simulink model "ADAS_Main"  (R2026a)
settings: Solver=FixedStepDiscrete  StopTime=5
InitFcn:
  | createLidarActorProfiles;
model workspace (MAT data in the model file):
  firstWarning = 1
  originalScenarioChecksum = '71EAF3DF157DF5A35F75811B676F8B0F'
undefined symbols (not defined in the file): driving, matlabshared
libraries: drivingscenarioandsensors x3, lidarlib x1
(part 1 of 6)
settings Model: Creator=sanga  LastModifiedBy=sanga
settings DebuggingCC: UnconnectedInputMsg=error

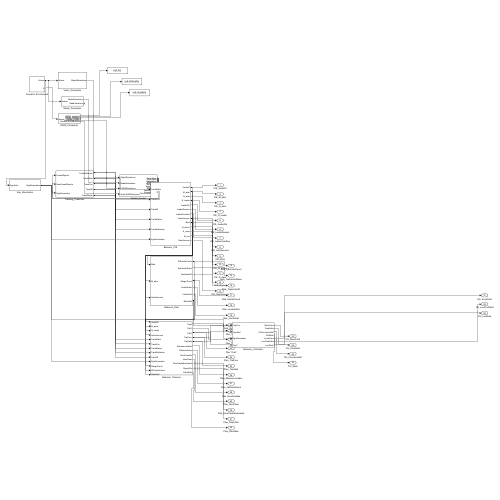
[thumbnail: Simulink's stored preview of the top-level diagram]
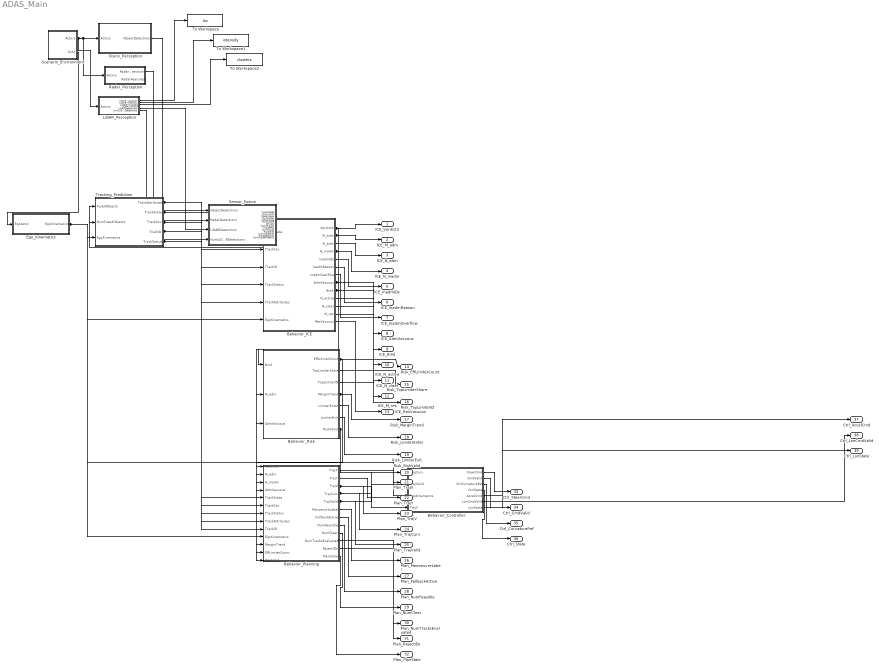
== system ADAS_Main ==
  Behavior_Controller : Subsystem
  Behavior_ICE : Subsystem
  Behavior_Planning : Subsystem
  Behavior_Risk : Subsystem
  Ego_Kinematics : Subsystem
  LiDAR_Perception : Subsystem
  Radar_Perception : Subsystem
  Scenario_Environment : Subsystem
  Sensor_Fusion : Subsystem
  To Workspace : ToWorkspace  VariableName=loc  SaveFormat=Timeseries  SampleTime=-1
  To Workspace1 : ToWorkspace  VariableName=intensity  SaveFormat=Timeseries  SampleTime=-1
  To Workspace2 : ToWorkspace  VariableName=clusters  SaveFormat=Timeseries  SampleTime=-1
  Tracking_Prediction : Subsystem
  Vision_Perception : Subsystem
  ICE_Verdict3 : Outport
  ICE_M_adm : Outport  Port=2
  ICE_N_adm : Outport  Port=3
  ICE_N_inadm : Outport  Port=4
  ICE_InadmIDs : Outport  Port=5
  ICE_InadmReason : Outport  Port=6
  ICE_InadmOverflow : Outport  Port=7
  ICE_AdmVacuous : Outport  Port=8
  ICE_Bind : Outport  Port=9
  ICE_N_active : Outport  Port=10
  ICE_N_clear : Outport  Port=11
  ICE_M_res : Outport  Port=12
  ICE_ResVacuous : Outport  Port=13
  Risk_EffLimiterCount : Outport  Port=14
  Risk_TopLimiterShare : Outport  Port=15
  Risk_TopLimiterID : Outport  Port=16
  Risk_MarginTrend : Outport  Port=17
  Risk_LimiterEnter : Outport  Port=18
  Risk_LimiterExit : Outport  Port=19
  Risk_RiskValid : Outport  Port=20
  Plan_TrajX : Outport  Port=21
  Plan_TrajY : Outport  Port=22
  Plan_TrajV : Outport  Port=23
  Plan_TrajCurv : Outport  Port=24
  Plan_TrajValid : Outport  Port=25
  Plan_ManoeuvreLabel : Outport  Port=26
  Plan_FallbackActive : Outport  Port=27
  Plan_NumFeasible : Outport  Port=28
  Plan_NumClear : Outport  Port=29
  Plan_NumTracksEvaluated : Outport  Port=30
  Plan_RejectIDs : Outport  Port=31
  Plan_PlanStale : Outport  Port=32
  Ctrl_SteerCmd : Outport  Port=33
  Ctrl_CmdValid : Outport  Port=34
  Ctrl_CurvatureRef : Outport  Port=35
  Ctrl_State : Outport  Port=36
  Ctrl_AccelCmd : Outport  Port=37
  Ctrl_LonCmdValid : Outport  Port=38
  Ctrl_LonState : Outport  Port=39
  wires:
  Scenario_Environment/1(Actors) -> Radar_Perception/1(Actors), Vision_Perception/1(Actors), LiDAR_Perception/1(Actors)
  LiDAR_Perception/1(LiDAR_Location) -> To Workspace/1
  LiDAR_Perception/2(LiDAR_Intensity) -> To Workspace1/1
  LiDAR_Perception/3(LiDAR_Clusters) -> To Workspace2/1
  Vision_Perception/1(ObjectDetections) -> Sensor_Fusion/1(ObjectDetections)
  Radar_Perception/1(RadarDetections) -> Sensor_Fusion/2(RadarDetections)
  LiDAR_Perception/5(LiDARDetections) -> Sensor_Fusion/3(LiDARDetections)
  LiDAR_Perception/6(NumLiDARDetections) -> Sensor_Fusion/4(NumLiDARDetections)
  Scenario_Environment/2(Out2) -> Ego_Kinematics/1(EgoActor)
  Sensor_Fusion/13(FusedObjects) -> Tracking_Prediction/1(FusedObjects)
  Sensor_Fusion/14(NumFusedObjects) -> Tracking_Prediction/2(NumFusedObjects)
  Ego_Kinematics/1(EgoKinematics) -> Tracking_Prediction/3(EgoKinematics), Behavior_ICE/6(EgoKinematics), Behavior_Planning/10(EgoKinematics), Behavior_Controller/3(EgoKinematics)
  Tracking_Prediction/2(TrackState) -> Behavior_ICE/1(TrackState), Behavior_Planning/5(TrackState)
  Tracking_Prediction/3(TrackCov) -> Behavior_ICE/2(TrackCov), Behavior_Planning/6(TrackCov)
  Tracking_Prediction/4(TrackID) -> Behavior_ICE/3(TrackID), Behavior_Planning/9(TrackID)
  Tracking_Prediction/5(TrackStatus) -> Behavior_ICE/4(TrackStatus), Behavior_Planning/7(TrackStatus)
  Tracking_Prediction/1(TrackAttributes) -> Behavior_ICE/5(TrackAttributes), Behavior_Planning/8(TrackAttributes)
  Behavior_ICE/1(Verdict3) -> ICE_Verdict3/1, Behavior_Planning/1(Verdict3)
  Behavior_ICE/2(M_adm) -> ICE_M_adm/1, Behavior_Risk/2(M_adm), Behavior_Planning/2(M_adm)
  Behavior_ICE/3(N_adm) -> ICE_N_adm/1
  Behavior_ICE/4(N_inadm) -> ICE_N_inadm/1, Behavior_Planning/3(N_inadm)
  Behavior_ICE/5(InadmIDs) -> ICE_InadmIDs/1
  Behavior_ICE/6(InadmReason) -> ICE_InadmReason/1
  Behavior_ICE/7(InadmOverflow) -> ICE_InadmOverflow/1
  Behavior_ICE/8(AdmVacuous) -> ICE_AdmVacuous/1, Behavior_Risk/3(AdmVacuous), Behavior_Planning/4(AdmVacuous)
  Behavior_ICE/9(Bind) -> ICE_Bind/1, Behavior_Risk/1(Bind)
  Behavior_ICE/10(N_active) -> ICE_N_active/1
  Behavior_ICE/11(N_clear) -> ICE_N_clear/1
  Behavior_ICE/12(M_res) -> ICE_M_res/1
  Behavior_ICE/13(ResVacuous) -> ICE_ResVacuous/1
  Behavior_Risk/1(EffLimiterCount) -> Risk_EffLimiterCount/1, Behavior_Planning/12(EffLimiterCount)
  Behavior_Risk/2(TopLimiterShare) -> Risk_TopLimiterShare/1
  Behavior_Risk/3(TopLimiterID) -> Risk_TopLimiterID/1
  Behavior_Risk/4(MarginTrend) -> Risk_MarginTrend/1, Behavior_Planning/11(MarginTrend)
  Behavior_Risk/5(LimiterEnter) -> Risk_LimiterEnter/1
  Behavior_Risk/6(LimiterExit) -> Risk_LimiterExit/1
  Behavior_Risk/7(RiskValid) -> Risk_RiskValid/1, Behavior_Planning/13(RiskValid)
  Behavior_Planning/1(TrajX) -> Plan_TrajX/1
  Behavior_Planning/2(TrajY) -> Plan_TrajY/1
  Behavior_Planning/3(TrajV) -> Plan_TrajV/1, Behavior_Controller/4(TrajV)
  Behavior_Planning/4(TrajCurv) -> Plan_TrajCurv/1, Behavior_Controller/1(TrajCurv)
  Behavior_Planning/5(TrajValid) -> Plan_TrajValid/1, Behavior_Controller/2(TrajValid)
  Behavior_Planning/6(ManoeuvreLabel) -> Plan_ManoeuvreLabel/1
  Behavior_Planning/7(FallbackActive) -> Plan_FallbackActive/1
  Behavior_Planning/8(NumFeasible) -> Plan_NumFeasible/1
  Behavior_Planning/9(NumClear) -> Plan_NumClear/1
  Behavior_Planning/10(NumTracksEvaluated) -> Plan_NumTracksEvaluated/1
  Behavior_Planning/11(RejectIDs) -> Plan_RejectIDs/1
  Behavior_Planning/12(PlanStale) -> Plan_PlanStale/1
  Behavior_Controller/1(SteerCmd) -> Ctrl_SteerCmd/1
  Behavior_Controller/2(CmdValid) -> Ctrl_CmdValid/1
  Behavior_Controller/3(CtrlCurvatureRef) -> Ctrl_CurvatureRef/1
  Behavior_Controller/4(CtrlState) -> Ctrl_State/1
  Behavior_Controller/5(AccelCmd) -> Ctrl_AccelCmd/1
  Behavior_Controller/6(LonCmdValid) -> Ctrl_LonCmdValid/1
  Behavior_Controller/7(LonState) -> Ctrl_LonState/1

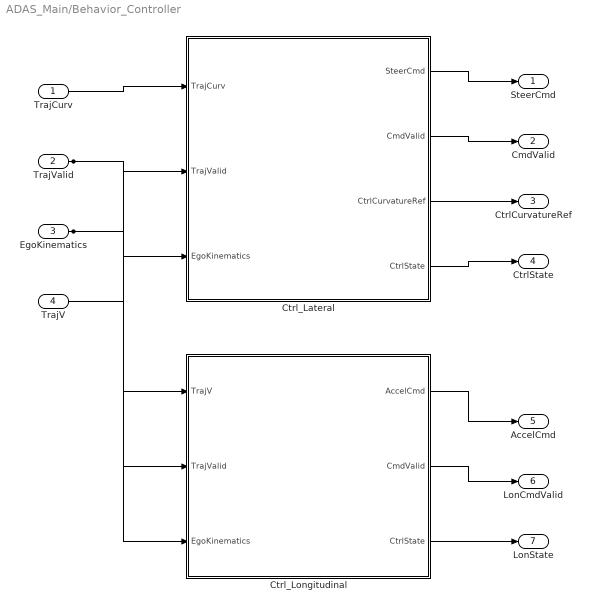
== system ADAS_Main/Behavior_Controller ==
  TrajCurv : Inport
  TrajValid : Inport  Port=2
  EgoKinematics : Inport  Port=3
  TrajV : Inport  Port=4
  Ctrl_Lateral : MATLAB Function  TreatAsAtomicUnit=on
  Ctrl_Longitudinal : MATLAB Function  TreatAsAtomicUnit=on
  SteerCmd : Outport
  CmdValid : Outport  Port=2
  CtrlCurvatureRef : Outport  Port=3
  CtrlState : Outport  Port=4
  AccelCmd : Outport  Port=5
  LonCmdValid : Outport  Port=6
  LonState : Outport  Port=7
  wires:
  TrajCurv/1 -> Ctrl_Lateral/1(TrajCurv)
  TrajValid/1 -> Ctrl_Lateral/2(TrajValid), Ctrl_Longitudinal/2(TrajValid)
  EgoKinematics/1 -> Ctrl_Lateral/3(EgoKinematics), Ctrl_Longitudinal/3(EgoKinematics)
  Ctrl_Lateral/1(SteerCmd) -> SteerCmd/1
  Ctrl_Lateral/2(CmdValid) -> CmdValid/1
  Ctrl_Lateral/3(CtrlCurvatureRef) -> CtrlCurvatureRef/1
  Ctrl_Lateral/4(CtrlState) -> CtrlState/1
  TrajV/1 -> Ctrl_Longitudinal/1(TrajV)
  Ctrl_Longitudinal/1(AccelCmd) -> AccelCmd/1
  Ctrl_Longitudinal/2(CmdValid) -> LonCmdValid/1
  Ctrl_Longitudinal/3(CtrlState) -> LonState/1

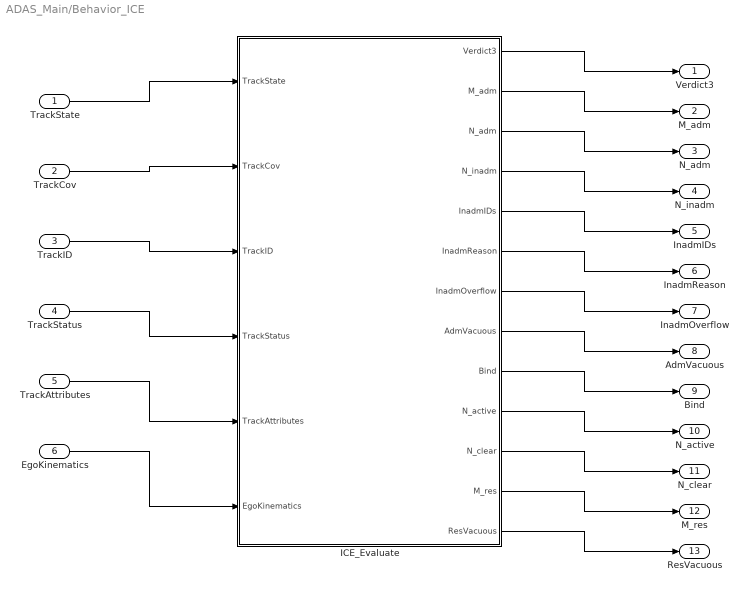
== system ADAS_Main/Behavior_ICE ==
  TrackState : Inport  OutDataTypeStr=double  PortDimensions=[512 4]
  TrackCov : Inport  Port=2  OutDataTypeStr=double  PortDimensions=[512 10]
  TrackID : Inport  Port=3  OutDataTypeStr=uint32  PortDimensions=[512 1]
  TrackStatus : Inport  Port=4  OutDataTypeStr=uint8  PortDimensions=[512 1]
  TrackAttributes : Inport  Port=5  OutDataTypeStr=double  PortDimensions=[512 4]
  EgoKinematics : Inport  Port=6  OutDataTypeStr=double  PortDimensions=[1 2]
  ICE_Evaluate : MATLAB Function  TreatAsAtomicUnit=on
  Verdict3 : Outport
  M_adm : Outport  Port=2
  N_adm : Outport  Port=3
  N_inadm : Outport  Port=4
  InadmIDs : Outport  Port=5
  InadmReason : Outport  Port=6
  InadmOverflow : Outport  Port=7
  AdmVacuous : Outport  Port=8
  Bind : Outport  Port=9
  N_active : Outport  Port=10
  N_clear : Outport  Port=11
  M_res : Outport  Port=12
  ResVacuous : Outport  Port=13
  wires:
  TrackState/1 -> ICE_Evaluate/1(TrackState)
  TrackCov/1 -> ICE_Evaluate/2(TrackCov)
  TrackID/1 -> ICE_Evaluate/3(TrackID)
  TrackStatus/1 -> ICE_Evaluate/4(TrackStatus)
  TrackAttributes/1 -> ICE_Evaluate/5(TrackAttributes)
  EgoKinematics/1 -> ICE_Evaluate/6(EgoKinematics)
  ICE_Evaluate/1(Verdict3) -> Verdict3/1
  ICE_Evaluate/2(M_adm) -> M_adm/1
  ICE_Evaluate/3(N_adm) -> N_adm/1
  ICE_Evaluate/4(N_inadm) -> N_inadm/1
  ICE_Evaluate/5(InadmIDs) -> InadmIDs/1
  ICE_Evaluate/6(InadmReason) -> InadmReason/1
  ICE_Evaluate/7(InadmOverflow) -> InadmOverflow/1
  ICE_Evaluate/8(AdmVacuous) -> AdmVacuous/1
  ICE_Evaluate/9(Bind) -> Bind/1
  ICE_Evaluate/10(N_active) -> N_active/1
  ICE_Evaluate/11(N_clear) -> N_clear/1
  ICE_Evaluate/12(M_res) -> M_res/1
  ICE_Evaluate/13(ResVacuous) -> ResVacuous/1

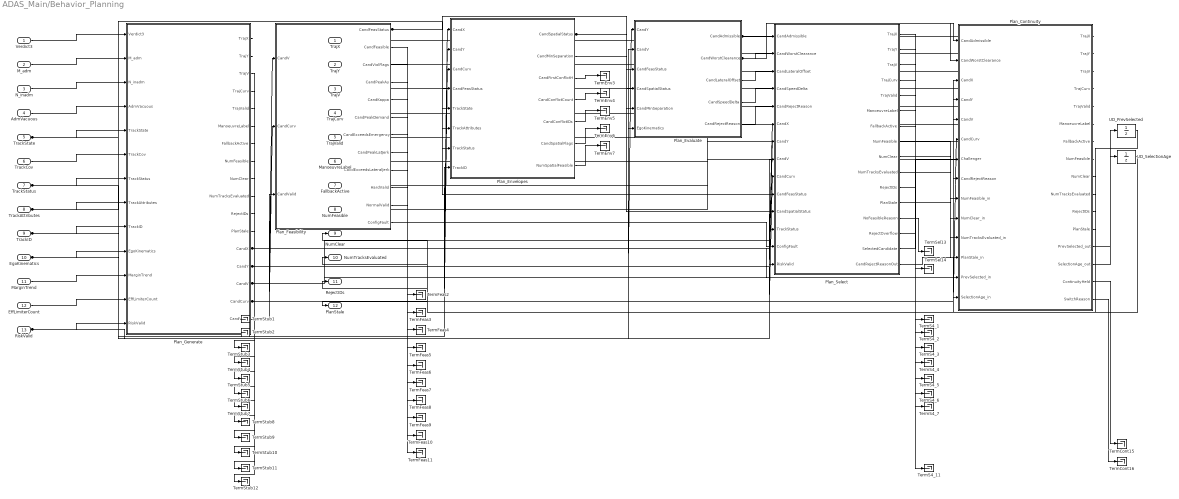
== system ADAS_Main/Behavior_Planning ==
  Verdict3 : Inport  OutDataTypeStr=int8  PortDimensions=[4 7]
  M_adm : Inport  Port=2  OutDataTypeStr=double  PortDimensions=[4 7]
  N_inadm : Inport  Port=3  OutDataTypeStr=uint16  PortDimensions=[1 1]
  AdmVacuous : Inport  Port=4  OutDataTypeStr=boolean  PortDimensions=[1 1]
  TrackState : Inport  Port=5  OutDataTypeStr=double  PortDimensions=[512 4]
  TrackCov : Inport  Port=6  OutDataTypeStr=double  PortDimensions=[512 10]
  TrackStatus : Inport  Port=7  OutDataTypeStr=uint8  PortDimensions=[512 1]
  TrackAttributes : Inport  Port=8  OutDataTypeStr=double  PortDimensions=[512 4]
  TrackID : Inport  Port=9  OutDataTypeStr=uint32  PortDimensions=[512 1]
  EgoKinematics : Inport  Port=10  OutDataTypeStr=double  PortDimensions=[1 2]
  MarginTrend : Inport  Port=11  OutDataTypeStr=double  PortDimensions=[4 7]
  EffLimiterCount : Inport  Port=12  OutDataTypeStr=double  PortDimensions=[4 1]
  RiskValid : Inport  Port=13  OutDataTypeStr=boolean  PortDimensions=[1 1]
  Plan_Continuity : MATLAB Function  TreatAsAtomicUnit=on
  Plan_Envelopes : MATLAB Function  TreatAsAtomicUnit=on
  Plan_Evaluate : MATLAB Function  TreatAsAtomicUnit=on
  Plan_Feasibility : MATLAB Function  TreatAsAtomicUnit=on
  Plan_Generate : MATLAB Function  TreatAsAtomicUnit=on
  Plan_Select : MATLAB Function  TreatAsAtomicUnit=on
  TermCont15 : Terminator
  TermCont16 : Terminator
  TermEnv{3..7} (5 alike) : Terminator
  TermFeas{2..11} (10 alike) : Terminator
  TermS4_{1..7,11} (8 alike) : Terminator
  TermSel13 : Terminator
  TermSel14 : Terminator
  TermStub{1..12} (12 alike) : Terminator
  UD_PrevSelected : UnitDelay  SampleTime=-1
  UD_SelectionAge : UnitDelay  SampleTime=-1
  TrajX : Outport
  TrajY : Outport  Port=2
  TrajV : Outport  Port=3
  TrajCurv : Outport  Port=4
  TrajValid : Outport  Port=5
  ManoeuvreLabel : Outport  Port=6
  FallbackActive : Outport  Port=7
  NumFeasible : Outport  Port=8
  NumClear : Outport  Port=9
  NumTracksEvaluated : Outport  Port=10
  RejectIDs : Outport  Port=11
  PlanStale : Outport  Port=12
  wires:
  Verdict3/1 -> Plan_Generate/1(Verdict3)
  M_adm/1 -> Plan_Generate/2(M_adm)
  N_inadm/1 -> Plan_Generate/3(N_inadm)
  AdmVacuous/1 -> Plan_Generate/4(AdmVacuous)
  TrackState/1 -> Plan_Generate/5(TrackState), Plan_Envelopes/5(TrackState)
  TrackCov/1 -> Plan_Generate/6(TrackCov)
  TrackStatus/1 -> Plan_Generate/7(TrackStatus), Plan_Envelopes/7(TrackStatus), Plan_Select/12(TrackStatus)
  TrackAttributes/1 -> Plan_Generate/8(TrackAttributes), Plan_Envelopes/6(TrackAttributes)
  TrackID/1 -> Plan_Generate/9(TrackID), Plan_Envelopes/8(TrackID)
  EgoKinematics/1 -> Plan_Generate/10(EgoKinematics), Plan_Evaluate/6(EgoKinematics)
  MarginTrend/1 -> Plan_Generate/11(MarginTrend)
  EffLimiterCount/1 -> Plan_Generate/12(EffLimiterCount)
  RiskValid/1 -> Plan_Generate/13(RiskValid), Plan_Select/14(RiskValid)
  Plan_Generate/15(CandV) -> Plan_Feasibility/1(CandV), Plan_Evaluate/2(CandV), Plan_Select/8(CandV), Plan_Continuity/5(CandV)
  Plan_Generate/16(CandCurv) -> Plan_Feasibility/2(CandCurv), Plan_Envelopes/3(CandCurv), Plan_Select/9(CandCurv), Plan_Continuity/6(CandCurv)
  Plan_Generate/17(CandValid) -> Plan_Feasibility/3(CandValid)
  Plan_Feasibility/2(CandFeasible) -> TermFeas2/1
  Plan_Feasibility/3(CandViolFlags) -> TermFeas3/1
  Plan_Feasibility/4(CandPeakAy) -> TermFeas4/1
  Plan_Feasibility/5(CandKappa) -> TermFeas5/1
  Plan_Feasibility/6(CandPeakDemand) -> TermFeas6/1
  Plan_Feasibility/7(CandExceedsEmergency) -> TermFeas7/1
  Plan_Feasibility/8(CandPeakLatJerk) -> TermFeas8/1
  Plan_Feasibility/9(CandExceedsLateralJerk) -> TermFeas9/1
  Plan_Feasibility/10(HardValid) -> TermFeas10/1
  Plan_Feasibility/11(NormalValid) -> TermFeas11/1
  Plan_Generate/13(CandX) -> Plan_Envelopes/1(CandX), Plan_Select/6(CandX), Plan_Continuity/3(CandX)
  Plan_Generate/14(CandY) -> Plan_Envelopes/2(CandY), Plan_Evaluate/1(CandY), Plan_Select/7(CandY), Plan_Continuity/4(CandY)
  Plan_Feasibility/1(CandFeasStatus) -> Plan_Envelopes/4(CandFeasStatus), Plan_Evaluate/3(CandFeasStatus), Plan_Select/10(CandFeasStatus)
  Plan_Envelopes/3(CandFirstConflictH) -> TermEnv3/1
  Plan_Envelopes/4(CandConflictCount) -> TermEnv4/1
  Plan_Envelopes/5(CandConflictIDs) -> TermEnv5/1
  Plan_Envelopes/6(CandSpatialFlags) -> TermEnv6/1
  Plan_Envelopes/7(NumSpatialFeasible) -> TermEnv7/1
  Plan_Generate/1(TrajX) -> TermStub1/1
  Plan_Generate/2(TrajY) -> TermStub2/1
  Plan_Generate/3(TrajV) -> TermStub3/1
  Plan_Generate/4(TrajCurv) -> TermStub4/1
  Plan_Generate/5(TrajValid) -> TermStub5/1
  Plan_Generate/6(ManoeuvreLabel) -> TermStub6/1
  Plan_Generate/7(FallbackActive) -> TermStub7/1
  Plan_Generate/8(NumFeasible) -> TermStub8/1
  Plan_Generate/9(NumClear) -> TermStub9/1
  Plan_Generate/10(NumTracksEvaluated) -> TermStub10/1
  Plan_Generate/11(RejectIDs) -> TermStub11/1
  Plan_Generate/12(PlanStale) -> TermStub12/1
  Plan_Envelopes/1(CandSpatialStatus) -> Plan_Evaluate/4(CandSpatialStatus), Plan_Select/11(CandSpatialStatus)
  Plan_Envelopes/2(CandMinSeparation) -> Plan_Evaluate/5(CandMinSeparation)
  Plan_Evaluate/1(CandAdmissible) -> Plan_Select/1(CandAdmissible), Plan_Continuity/1(CandAdmissible)
  Plan_Evaluate/2(CandWorstClearance) -> Plan_Select/2(CandWorstClearance), Plan_Continuity/2(CandWorstClearance)
  Plan_Evaluate/3(CandLateralOffset) -> Plan_Select/3(CandLateralOffset)
  Plan_Evaluate/4(CandSpeedDelta) -> Plan_Select/4(CandSpeedDelta)
  Plan_Evaluate/5(CandRejectReason) -> Plan_Select/5(CandRejectReason)
  Plan_Feasibility/12(ConfigFault) -> Plan_Select/13(ConfigFault)
  Plan_Select/13(NoFeasibleReason) -> TermSel13/1
  Plan_Select/14(RejectOverflow) -> TermSel14/1
  Plan_Select/15(SelectedCandidate) -> Plan_Continuity/7(Challenger)
  Plan_Select/16(CandRejectReasonOut) -> Plan_Continuity/8(CandRejectReason)
  Plan_Select/8(NumFeasible) -> Plan_Continuity/9(NumFeasible_in)
  Plan_Select/9(NumClear) -> Plan_Continuity/10(NumClear_in)
  Plan_Select/10(NumTracksEvaluated) -> Plan_Continuity/11(NumTracksEvaluated_in)
  Plan_Select/12(PlanStale) -> Plan_Continuity/12(PlanStale_in)
  UD_PrevSelected/1 -> Plan_Continuity/13(PrevSelected_in)
  UD_SelectionAge/1 -> Plan_Continuity/14(SelectionAge_in)
  Plan_Continuity/1(TrajX) -> TrajX/1
  Plan_Continuity/2(TrajY) -> TrajY/1
  Plan_Continuity/3(TrajV) -> TrajV/1
  Plan_Continuity/4(TrajCurv) -> TrajCurv/1
  Plan_Continuity/5(TrajValid) -> TrajValid/1
  Plan_Continuity/6(ManoeuvreLabel) -> ManoeuvreLabel/1
  Plan_Continuity/7(FallbackActive) -> FallbackActive/1
  Plan_Continuity/8(NumFeasible) -> NumFeasible/1
  Plan_Continuity/9(NumClear) -> NumClear/1
  Plan_Continuity/10(NumTracksEvaluated) -> NumTracksEvaluated/1
  Plan_Continuity/11(RejectIDs) -> RejectIDs/1
  Plan_Continuity/12(PlanStale) -> PlanStale/1
  Plan_Continuity/13(PrevSelected_out) -> UD_PrevSelected/1
  Plan_Continuity/14(SelectionAge_out) -> UD_SelectionAge/1
  Plan_Continuity/15(ContinuityHeld) -> TermCont15/1
  Plan_Continuity/16(SwitchReason) -> TermCont16/1
  Plan_Select/1(TrajX) -> TermS4_1/1
  Plan_Select/2(TrajY) -> TermS4_2/1
  Plan_Select/3(TrajV) -> TermS4_3/1
  Plan_Select/4(TrajCurv) -> TermS4_4/1
  Plan_Select/5(TrajValid) -> TermS4_5/1
  Plan_Select/6(ManoeuvreLabel) -> TermS4_6/1
  Plan_Select/7(FallbackActive) -> TermS4_7/1
  Plan_Select/11(RejectIDs) -> TermS4_11/1

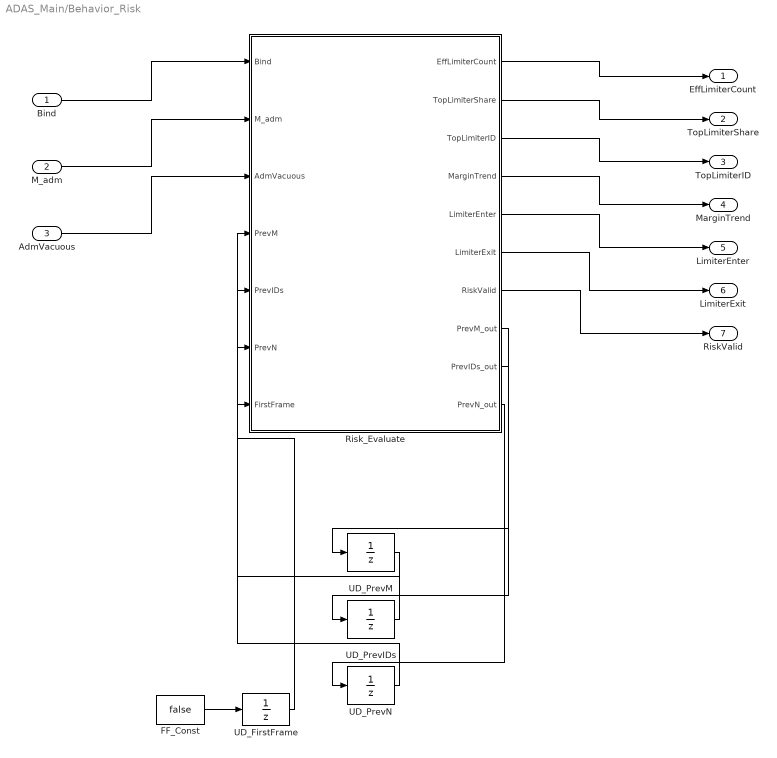
== system ADAS_Main/Behavior_Risk ==
  Bind : Inport  OutDataTypeStr=uint32  PortDimensions=[4 7 8]
  M_adm : Inport  Port=2  OutDataTypeStr=double  PortDimensions=[4 7]
  AdmVacuous : Inport  Port=3  OutDataTypeStr=boolean  PortDimensions=[1 1]
  FF_Const : Constant  Value=false  OutDataTypeStr=boolean
  Risk_Evaluate : MATLAB Function  TreatAsAtomicUnit=on
  UD_FirstFrame : UnitDelay  InitialCondition=1  SampleTime=0.1
  UD_PrevIDs : UnitDelay  SampleTime=0.1
  UD_PrevM : UnitDelay  SampleTime=0.1
  UD_PrevN : UnitDelay  SampleTime=0.1
  EffLimiterCount : Outport
  TopLimiterShare : Outport  Port=2
  TopLimiterID : Outport  Port=3
  MarginTrend : Outport  Port=4
  LimiterEnter : Outport  Port=5
  LimiterExit : Outport  Port=6
  RiskValid : Outport  Port=7
  wires:
  Bind/1 -> Risk_Evaluate/1(Bind)
  M_adm/1 -> Risk_Evaluate/2(M_adm)
  AdmVacuous/1 -> Risk_Evaluate/3(AdmVacuous)
  Risk_Evaluate/8(PrevM_out) -> UD_PrevM/1
  UD_PrevM/1 -> Risk_Evaluate/4(PrevM)
  Risk_Evaluate/9(PrevIDs_out) -> UD_PrevIDs/1
  UD_PrevIDs/1 -> Risk_Evaluate/5(PrevIDs)
  Risk_Evaluate/10(PrevN_out) -> UD_PrevN/1
  UD_PrevN/1 -> Risk_Evaluate/6(PrevN)
  FF_Const/1 -> UD_FirstFrame/1
  UD_FirstFrame/1 -> Risk_Evaluate/7(FirstFrame)
  Risk_Evaluate/1(EffLimiterCount) -> EffLimiterCount/1
  Risk_Evaluate/2(TopLimiterShare) -> TopLimiterShare/1
  Risk_Evaluate/3(TopLimiterID) -> TopLimiterID/1
  Risk_Evaluate/4(MarginTrend) -> MarginTrend/1
  Risk_Evaluate/5(LimiterEnter) -> LimiterEnter/1
  Risk_Evaluate/6(LimiterExit) -> LimiterExit/1
  Risk_Evaluate/7(RiskValid) -> RiskValid/1

== system ADAS_Main/Ego_Kinematics ==
  EgoActor : Inport
  Extract_Ego_Kinematics : MATLAB Function  TreatAsAtomicUnit=on
  TW_EgoKin : ToWorkspace  VariableName=egoKin  SaveFormat=Timeseries  SampleTime=-1
  EgoKinematics : Outport
  wires:
  EgoActor/1 -> Extract_Ego_Kinematics/1(egoActor)
  Extract_Ego_Kinematics/1(egoKin) -> EgoKinematics/1, TW_EgoKin/1

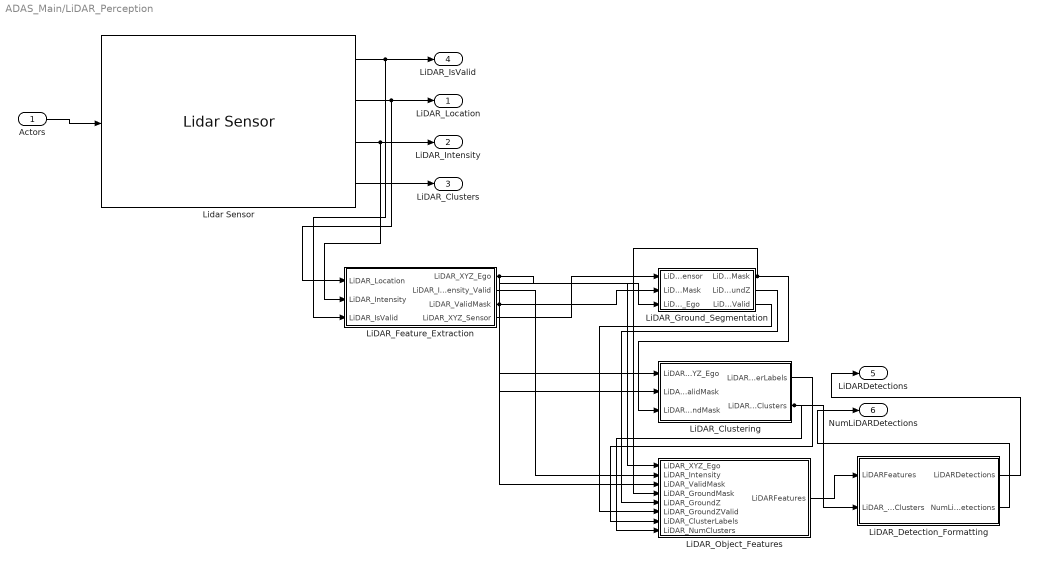
== system ADAS_Main/LiDAR_Perception ==
  Actors : Inport
  LiDAR_Clustering : Subsystem
  LiDAR_Detection_Formatting : Subsystem
  LiDAR_Feature_Extraction : Subsystem
  LiDAR_Ground_Segmentation : Subsystem
  LiDAR_Object_Features : Subsystem
  Lidar Sensor : lidarlib/Lidar Sensor  SensorIndex=1  UpdateRate=0.1  Model=Custom  SensorPosition=[1.5 0 1.6]  SensorOrientation=[0 0 0]  ActorProfilesVariableName=actor_profiles  HostID=1  CoordinateSystem=Sensor  MaxRange=120  AzimuthLimits=[-180 180]  AzimuthResolution=0.16  UseCustomElevationAngles=off  ElevationAngles=[-25 -15.6 -11.3 -8.8:0.9:-4 -4:0.32:1.6 3.3 4.6 7 10.3 15]  ElevationLimits=[-20 20]  ElevationResolution=0.4  HasNoise=on  RangeAccuracy=0.01  FogVisibility=1000  Rainrate=0  HasMotionDistortion=off  FiringTimes=[]  MaterialAttributesJSON=|  EditMaterialAttributesJSON=off  OutputIntensity=on  OutputClusters=on
      | [
      | {"Material":"Aluminum","Reflectance":0.63,"Diffuseness":1,"Roughness":0.3,"Description":"Weathered aluminum metal from roof"},
      | {"Material":"Asphalt","Reflectance":0.1,"Diffuseness":1,"Roughness":0.3,"Description":"Road or construction material"},
      | {"Material":"Bark","Reflectance":0.56,"Diffuseness":1,"Roughness":0.3,"Description":"Pinus ponderosa tree bark"},
      | {"Material":"Brick","Reflectance":0.29,"Diffuseness":1,"Roughness":0.3,"Description":"Smooth-faced red building construction brick"},
      | {"Material":"Cement","Reflectance":0.35,"Diffuseness":1,"Roughness":0.3,"Description":"Cement construction concrete cinderblock"},
      | {"Material":"Concrete","Reflectance":0.33,"Diffuseness":1,"Roughness":0.3,"Description":"Road or construction material"},
      | {"Material":"Copper","Reflectance":0.57,"Diffuseness":1,"Roughness":0.3,"Description":"Weathered copper metal from roof"},
      | {"Material":"Default","Reflectance":1,"Diffuseness":1,"Roughness":0.3,"Description":"Default material attributes"},
      | {"Material":"Glass","Reflectance":0.08,"Diffuseness":1,"Roughness":0.3,"Description":"Transparent construction plate window glass"},
      | {"Material":"Grass","Reflectance":0.5,"Diffuseness":1,"Roughness":0.3,"Description":"Green Rye grass"},
      | {"Material":"Ice","Reflectance":0.017,"Diffuseness":1,"Roughness":0.3,"Description":"Ice"},
      | {"Material":"Leaves","Reflectance":0.56,"Diffuseness":1,"Roughness":0.3,"Description":"Quercus species (Oak tree) leaves"},
      | {"Material":"Marble","Reflectance":0.84,"Diffuseness":1,"Roughness":0.3,"Description":"White weathered construction marble"},
      | {"Material":"Rubber","Reflectance":0.6,"Diffuseness":1,"Roughness":0.3,"Description":"White rubberized coating from building roof"},
      | {"Material":"Snow","Reflectance":0.71,"Diffuseness":1,"Roughness":0.3,"Description":"Coarse granular snow"},
      | {"Material":"Steel","Reflectance":0.064,"Diffuseness":1,"Roughness":0.3,"Description":"Weathered, galvanized steel metal from roof"},
      | {"Material":"Tar","Reflectance":0.07,"Diffuseness":1,"Roughness":0.3,"Description":"Black, glossy construction tar"},
      | {"Material":"Terracotta","Reflectance":0.17,"Diffuseness":1,"Roughness":0.3,"Description":"Weathered terra cotta roofing tile of ceramic composite construction"},
      | {"Material":"Water","Reflectance":0.025,"Diffuseness":1,"Roughness":0.3,"Description":"Tap water"},
      | {"Material":"Wood","Reflectance":0.85,"Diffuseness":1,"Roughness":0.3,"Description":"Bare pine wood construction lumber"}
      | ]
  LiDAR_Location : Outport
  LiDAR_Intensity : Outport  Port=2
  LiDAR_Clusters : Outport  Port=3
  LiDAR_IsValid : Outport  Port=4
  LiDARDetections : Outport  Port=5
  NumLiDARDetections : Outport  Port=6
  wires:
  Lidar Sensor/2 -> LiDAR_Feature_Extraction/1(LiDAR_Location), LiDAR_Location/1
  Lidar Sensor/3 -> LiDAR_Feature_Extraction/2(LiDAR_Intensity), LiDAR_Intensity/1
  Lidar Sensor/4 -> LiDAR_Clusters/1
  Lidar Sensor/1 -> LiDAR_Feature_Extraction/3(LiDAR_IsValid), LiDAR_IsValid/1
  LiDAR_Feature_Extraction/4(LiDAR_XYZ_Sensor) -> LiDAR_Ground_Segmentation/1(LiDAR_XYZ_Sensor)
  LiDAR_Feature_Extraction/3(LiDAR_ValidMask) -> LiDAR_Ground_Segmentation/2(LiDAR_ValidMask), LiDAR_Clustering/2(LiDAR_ValidMask), LiDAR_Object_Features/3(LiDAR_ValidMask)
  Actors/1 -> Lidar Sensor/1
  LiDAR_Feature_Extraction/1(LiDAR_XYZ_Ego) -> LiDAR_Ground_Segmentation/3(LiDAR_XYZ_Ego), LiDAR_Clustering/1(LiDAR_XYZ_Ego), LiDAR_Object_Features/1(LiDAR_XYZ_Ego)
  LiDAR_Ground_Segmentation/1(LiDAR_GroundMask) -> LiDAR_Clustering/3(LiDAR_GroundMask), LiDAR_Object_Features/4(LiDAR_GroundMask)
  LiDAR_Feature_Extraction/2(LiDAR_Intensity_Valid) -> LiDAR_Object_Features/2(LiDAR_Intensity)
  LiDAR_Ground_Segmentation/2(LiDAR_GroundZ) -> LiDAR_Object_Features/5(LiDAR_GroundZ)
  LiDAR_Ground_Segmentation/3(LiDAR_GroundZValid) -> LiDAR_Object_Features/6(LiDAR_GroundZValid)
  LiDAR_Clustering/1(LiDAR_ClusterLabels) -> LiDAR_Object_Features/7(LiDAR_ClusterLabels)
  LiDAR_Clustering/2(LiDAR_NumClusters) -> LiDAR_Object_Features/8(LiDAR_NumClusters), LiDAR_Detection_Formatting/2(LiDAR_NumClusters)
  LiDAR_Object_Features/1(LiDARFeatures) -> LiDAR_Detection_Formatting/1(LiDARFeatures)
  LiDAR_Detection_Formatting/1(LiDARDetections) -> LiDARDetections/1
  LiDAR_Detection_Formatting/2(NumLiDARDetections) -> NumLiDARDetections/1

== system ADAS_Main/Radar_Perception ==
  Actors : Inport
  Driving Radar Data Generator : drivingscenarioandsensors/Driving Radar Data Generator  SensorIndex=2  UpdateRate=10  MountingLocation=[ 3.4, 0, 0.2 ]  MountingAngles=[0 0 0]  HasElevation=off  HasRangeRate=on  HasNoise=on  HasFalseAlarms=on  HasOcclusion=on  MaxNumReportsSource=Property  MaxNumReports=50  TargetReportFormat=Clustered detections  DetectionCoordinates=Body  TrackCoordinates=Body  BusNameSource=Auto  BusName=BusDrivingRadarDataGenerator  SimulateUsing=Interpreted execution  AzimuthResolution=4  ElevationResolution=5  RangeResolution=2.5  RangeRateResolution=0.5  AzimuthBiasFraction=0.1  ElevationBiasFraction=0.1  RangeBiasFraction=0.05  RangeRateBiasFraction=0.05  FieldOfView=[ 20, 5 ]  RangeLimits=[ 0, 150 ]  RangeRateLimits=[ -100, 100 ]  DetectionProbability=0.9  FalseAlarmRate=1e-06  ReferenceRange=100  ReferenceRCS=0  CenterFrequency=77e9  FilterInitializationFcn=initcvekf  ConfirmationThreshold=[2 3]  DeletionThreshold=[5 5]  InitialSeedSource=Repeatable  InitialSeed=0  UsedSeed=matlabshared.tracking.internal.SimulinkUtilities.seedManager(gcb)  ProfilesSource=From Scenario Reader block  ProfilesParameters=driving.internal.ActorProfilesRadarParameters  ProfilesExpression=struct('ClassID',0,'Length',4.7,'Width',1.8,'Height',1.4,'OriginOffset',[-1.35 0 0],'RCSPattern',[10 10;10 10],'RCSAzimuthAngles',[-180 180],'RCSElevationAngles',[-90 90])
  Radar_Feature_Extraction : Subsystem
  RadarDetections : Outport
  RadarFeatures : Outport  Port=2
  wires:
  Actors/1 -> Driving Radar Data Generator/1
  Driving Radar Data Generator/1 -> Radar_Feature_Extraction/1(RawRadarDetections)
  Radar_Feature_Extraction/1(EnhancedRadar) -> RadarDetections/1
  Radar_Feature_Extraction/2(RadarFeatures) -> RadarFeatures/1

== system ADAS_Main/Scenario_Environment ==
  Bus Selector : BusSelector  OutputSignals=Position,Velocity
  Scenario Reader : drivingscenarioandsensors/Scenario Reader  Priority=-1  ScenarioSource=From file  ScenarioFileName=D:\AutonomousDriving\D_scenarios\V2_0_CameraScenario.mat  ScenarioVariableName=scenario  OutputCoordinateSystem=Vehicle coordinates  EgoVehicleSource=Scenario  EgoVehicleActorID=1  OrientVehiclesOnRoad=off  OutputEgoVehiclePose=on  OutputEgoVehicleState=on  SampleTime=0.1  LaneBoundaryOutput=None  LaneBoundaryDistance=0:0.5:9.5  LaneBoundaryLocation=Center of lane markings  BusNameSource=Auto  BusName=BusActors  BusNumActorsSource=Scenario  BusNumActors=100  BusName2Source=Auto  BusName2=BusLaneBoundaries  BusNumLaneBoundariesSource=Scenario  BusNumLaneBoundaries=10  BusName3Source=Auto  BusName3=BusEgoActor  BusName4Source=Auto  BusName4=BusEgoState  ShowCoordinateLabels=on  SimulateUsing=Interpreted execution
  Scope : Scope
      settings: ActiveDisplayYMinimum=-16.478455804620214  ActiveDisplayYMaximum=59.403600827046532
  Scope1 : Scope
      settings: ActiveDisplayYMinimum=-0.75912369165439664  ActiveDisplayYMaximum=11.206530935880661
  Actors : Outport
  Out2 : Outport  Port=2
  wires:
  Bus Selector/2 -> Scope1/1  "<Velocity>"
  Scenario Reader/3 -> Bus Selector/1
  Scenario Reader/1 -> Actors/1
  Scenario Reader/2 -> Out2/1
  Bus Selector/1 -> Scope/1  "<Position>"

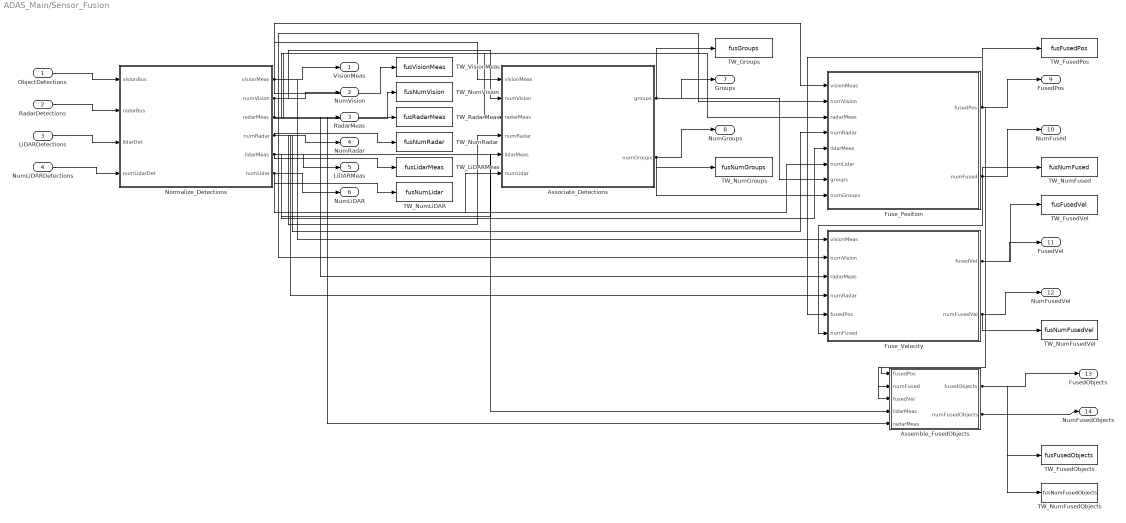
== system ADAS_Main/Sensor_Fusion ==
  ObjectDetections : Inport
  RadarDetections : Inport  Port=2
  LiDARDetections : Inport  Port=3
  NumLiDARDetections : Inport  Port=4
  Assemble_FusedObjects : MATLAB Function  TreatAsAtomicUnit=on
  Associate_Detections : MATLAB Function  TreatAsAtomicUnit=on
  Fuse_Position : MATLAB Function  TreatAsAtomicUnit=on
  Fuse_Velocity : MATLAB Function  TreatAsAtomicUnit=on
  Normalize_Detections : MATLAB Function  TreatAsAtomicUnit=on
  TW_FusedObjects : ToWorkspace  VariableName=fusFusedObjects  SaveFormat=Timeseries  SampleTime=-1
  TW_FusedPos : ToWorkspace  VariableName=fusFusedPos  SaveFormat=Timeseries  SampleTime=-1
  TW_FusedVel : ToWorkspace  VariableName=fusFusedVel  SaveFormat=Timeseries  SampleTime=-1
  TW_Groups : ToWorkspace  VariableName=fusGroups  SaveFormat=Timeseries  SampleTime=-1
  TW_LiDARMeas : ToWorkspace  VariableName=fusLidarMeas  SaveFormat=Timeseries  SampleTime=-1
  TW_NumFused : ToWorkspace  VariableName=fusNumFused  SaveFormat=Timeseries  SampleTime=-1
  TW_NumFusedObjects : ToWorkspace  VariableName=fusNumFusedObjects  SaveFormat=Timeseries  SampleTime=-1
  TW_NumFusedVel : ToWorkspace  VariableName=fusNumFusedVel  SaveFormat=Timeseries  SampleTime=-1
  TW_NumGroups : ToWorkspace  VariableName=fusNumGroups  SaveFormat=Timeseries  SampleTime=-1
  TW_NumLiDAR : ToWorkspace  VariableName=fusNumLidar  SaveFormat=Timeseries  SampleTime=-1
  TW_NumRadar : ToWorkspace  VariableName=fusNumRadar  SaveFormat=Timeseries  SampleTime=-1
  TW_NumVision : ToWorkspace  VariableName=fusNumVision  SaveFormat=Timeseries  SampleTime=-1
  TW_RadarMeas : ToWorkspace  VariableName=fusRadarMeas  SaveFormat=Timeseries  SampleTime=-1
  TW_VisionMeas : ToWorkspace  VariableName=fusVisionMeas  SaveFormat=Timeseries  SampleTime=-1
  VisionMeas : Outport
  NumVision : Outport  Port=2
  RadarMeas : Outport  Port=3
  NumRadar : Outport  Port=4
  LiDARMeas : Outport  Port=5
  NumLiDAR : Outport  Port=6
  Groups : Outport  Port=7
  NumGroups : Outport  Port=8
  FusedPos : Outport  Port=9
  NumFused : Outport  Port=10
  FusedVel : Outport  Port=11
  NumFusedVel : Outport  Port=12
  FusedObjects : Outport  Port=13
  NumFusedObjects : Outport  Port=14
  wires:
  ObjectDetections/1 -> Normalize_Detections/1(visionBus)
  RadarDetections/1 -> Normalize_Detections/2(radarBus)
  LiDARDetections/1 -> Normalize_Detections/3(lidarDet)
  NumLiDARDetections/1 -> Normalize_Detections/4(numLidarDet)
  Normalize_Detections/1(visionMeas) -> VisionMeas/1, TW_VisionMeas/1, Associate_Detections/1(visionMeas), Fuse_Position/1(visionMeas), Fuse_Velocity/1(visionMeas)
  Normalize_Detections/2(numVision) -> NumVision/1, TW_NumVision/1, Associate_Detections/2(numVision), Fuse_Position/2(numVision), Fuse_Velocity/2(numVision)
  Normalize_Detections/3(radarMeas) -> RadarMeas/1, TW_RadarMeas/1, Associate_Detections/3(radarMeas), Fuse_Position/3(radarMeas), Fuse_Velocity/3(radarMeas), Assemble_FusedObjects/5(radarMeas)
  Normalize_Detections/4(numRadar) -> NumRadar/1, TW_NumRadar/1, Associate_Detections/4(numRadar), Fuse_Position/4(numRadar), Fuse_Velocity/4(numRadar)
  Normalize_Detections/5(lidarMeas) -> LiDARMeas/1, TW_LiDARMeas/1, Associate_Detections/5(lidarMeas), Fuse_Position/5(lidarMeas), Assemble_FusedObjects/4(lidarMeas)
  Normalize_Detections/6(numLidar) -> NumLiDAR/1, TW_NumLiDAR/1, Associate_Detections/6(numLidar), Fuse_Position/6(numLidar)
  Associate_Detections/1(groups) -> Groups/1, TW_Groups/1, Fuse_Position/7(groups)
  Associate_Detections/2(numGroups) -> NumGroups/1, TW_NumGroups/1, Fuse_Position/8(numGroups)
  Fuse_Position/1(fusedPos) -> FusedPos/1, TW_FusedPos/1, Fuse_Velocity/5(fusedPos), Assemble_FusedObjects/1(fusedPos)
  Fuse_Position/2(numFused) -> NumFused/1, TW_NumFused/1, Fuse_Velocity/6(numFused), Assemble_FusedObjects/2(numFused)
  Fuse_Velocity/1(fusedVel) -> FusedVel/1, TW_FusedVel/1, Assemble_FusedObjects/3(fusedVel)
  Fuse_Velocity/2(numFusedVel) -> NumFusedVel/1, TW_NumFusedVel/1
  Assemble_FusedObjects/1(fusedObjects) -> FusedObjects/1, TW_FusedObjects/1
  Assemble_FusedObjects/2(numFusedObjects) -> NumFusedObjects/1, TW_NumFusedObjects/1

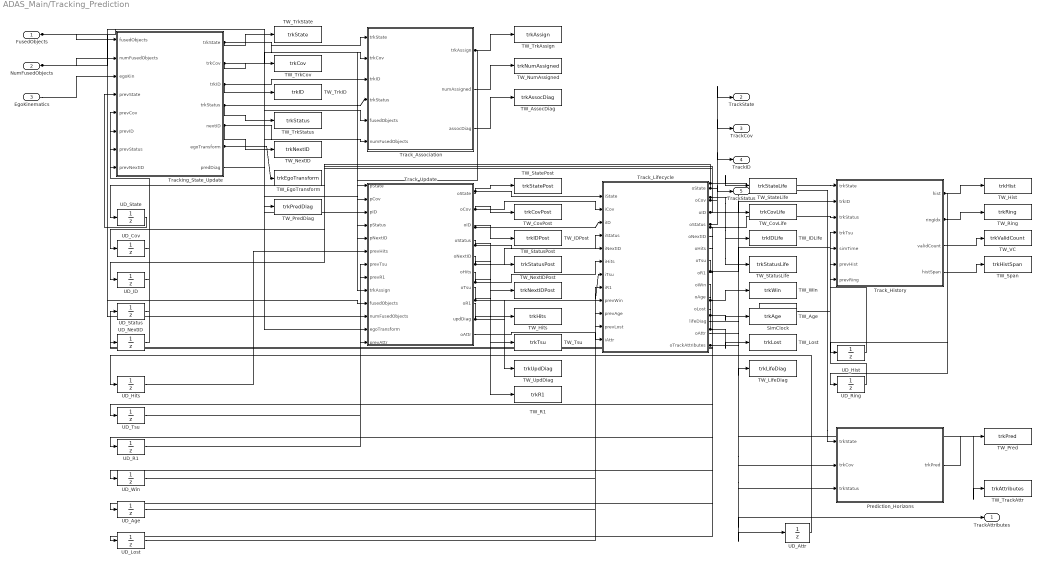
== system ADAS_Main/Tracking_Prediction ==
  FusedObjects : Inport
  NumFusedObjects : Inport  Port=2
  EgoKinematics : Inport  Port=3
  Prediction_Horizons : MATLAB Function  TreatAsAtomicUnit=on
  SimClock : DigitalClock  SampleTime=0.1
  TW_Age : ToWorkspace  VariableName=trkAge  SaveFormat=Timeseries  SampleTime=-1
  TW_AssocDiag : ToWorkspace  VariableName=trkAssocDiag  SaveFormat=Timeseries  SampleTime=-1
  TW_CovLife : ToWorkspace  VariableName=trkCovLife  SaveFormat=Timeseries  SampleTime=-1
  TW_CovPost : ToWorkspace  VariableName=trkCovPost  SaveFormat=Timeseries  SampleTime=-1
  TW_EgoTransform : ToWorkspace  VariableName=trkEgoTransform  SaveFormat=Timeseries  SampleTime=-1
  TW_Hist : ToWorkspace  VariableName=trkHist  SaveFormat=Timeseries  SampleTime=-1
  TW_Hits : ToWorkspace  VariableName=trkHits  SaveFormat=Timeseries  SampleTime=-1
  TW_IDLife : ToWorkspace  VariableName=trkIDLife  SaveFormat=Timeseries  SampleTime=-1
  TW_IDPost : ToWorkspace  VariableName=trkIDPost  SaveFormat=Timeseries  SampleTime=-1
  TW_LifeDiag : ToWorkspace  VariableName=trkLifeDiag  SaveFormat=Timeseries  SampleTime=-1
  TW_Lost : ToWorkspace  VariableName=trkLost  SaveFormat=Timeseries  SampleTime=-1
  TW_NextID : ToWorkspace  VariableName=trkNextID  SaveFormat=Timeseries  SampleTime=-1
  TW_NextIDPost : ToWorkspace  VariableName=trkNextIDPost  SaveFormat=Timeseries  SampleTime=-1
  TW_NumAssigned : ToWorkspace  VariableName=trkNumAssigned  SaveFormat=Timeseries  SampleTime=-1
  TW_Pred : ToWorkspace  VariableName=trkPred  SaveFormat=Timeseries  SampleTime=-1
  TW_PredDiag : ToWorkspace  VariableName=trkPredDiag  SaveFormat=Timeseries  SampleTime=-1
  TW_R1 : ToWorkspace  VariableName=trkR1  SaveFormat=Timeseries  SampleTime=-1
  TW_Ring : ToWorkspace  VariableName=trkRing  SaveFormat=Timeseries  SampleTime=-1
  TW_Span : ToWorkspace  VariableName=trkHistSpan  SaveFormat=Timeseries  SampleTime=-1
  TW_StateLife : ToWorkspace  VariableName=trkStateLife  SaveFormat=Timeseries  SampleTime=-1
  TW_StatePost : ToWorkspace  VariableName=trkStatePost  SaveFormat=Timeseries  SampleTime=-1
  TW_StatusLife : ToWorkspace  VariableName=trkStatusLife  SaveFormat=Timeseries  SampleTime=-1
  TW_StatusPost : ToWorkspace  VariableName=trkStatusPost  SaveFormat=Timeseries  SampleTime=-1
  TW_TrackAttr : ToWorkspace  VariableName=trkAttributes  SaveFormat=Timeseries  SampleTime=-1
  TW_TrkAssign : ToWorkspace  VariableName=trkAssign  SaveFormat=Timeseries  SampleTime=-1
  TW_TrkCov : ToWorkspace  VariableName=trkCov  SaveFormat=Timeseries  SampleTime=-1
  TW_TrkID : ToWorkspace  VariableName=trkID  SaveFormat=Timeseries  SampleTime=-1
  TW_TrkState : ToWorkspace  VariableName=trkState  SaveFormat=Timeseries  SampleTime=-1
  TW_TrkStatus : ToWorkspace  VariableName=trkStatus  SaveFormat=Timeseries  SampleTime=-1
  TW_Tsu : ToWorkspace  VariableName=trkTsu  SaveFormat=Timeseries  SampleTime=-1
  TW_UpdDiag : ToWorkspace  VariableName=trkUpdDiag  SaveFormat=Timeseries  SampleTime=-1
  TW_VC : ToWorkspace  VariableName=trkValidCount  SaveFormat=Timeseries  SampleTime=-1
  TW_Win : ToWorkspace  VariableName=trkWin  SaveFormat=Timeseries  SampleTime=-1
  Track_Association : MATLAB Function  TreatAsAtomicUnit=on
  Track_History : MATLAB Function  TreatAsAtomicUnit=on
  Track_Lifecycle : MATLAB Function  TreatAsAtomicUnit=on
  Track_Update : MATLAB Function  TreatAsAtomicUnit=on
  Tracking_State_Update : MATLAB Function  TreatAsAtomicUnit=on
  UD_Age : UnitDelay  SampleTime=0.1
  UD_Attr : UnitDelay  SampleTime=-1
  UD_Cov : UnitDelay  SampleTime=0.1
  UD_Hist : UnitDelay  SampleTime=0.1
  UD_Hits : UnitDelay  SampleTime=0.1
  UD_ID : UnitDelay  SampleTime=0.1
  UD_Lost : UnitDelay  SampleTime=0.1
  UD_NextID : UnitDelay  InitialCondition=1  SampleTime=0.1
  UD_R1 : UnitDelay  SampleTime=0.1
  UD_Ring : UnitDelay  SampleTime=0.1
  UD_State : UnitDelay  SampleTime=0.1
  UD_Status : UnitDelay  SampleTime=0.1
  UD_Tsu : UnitDelay  SampleTime=0.1
  UD_Win : UnitDelay  SampleTime=0.1
  TrackAttributes : Outport
  TrackState : Outport  Port=2
  TrackCov : Outport  Port=3
  TrackID : Outport  Port=4
  TrackStatus : Outport  Port=5
  wires:
  FusedObjects/1 -> Tracking_State_Update/1(fusedObjects), Track_Association/5(fusedObjects), Track_Update/10(fusedObjects)
  NumFusedObjects/1 -> Tracking_State_Update/2(numFusedObjects), Track_Association/6(numFusedObjects), Track_Update/11(numFusedObjects)
  EgoKinematics/1 -> Tracking_State_Update/3(egoKin)
  Tracking_State_Update/1(trkState) -> Track_Association/1(trkState), TW_TrkState/1, Track_Update/1(pState)
  UD_State/1 -> Tracking_State_Update/4(prevState)
  Tracking_State_Update/2(trkCov) -> Track_Association/2(trkCov), TW_TrkCov/1, Track_Update/2(pCov)
  UD_Cov/1 -> Tracking_State_Update/5(prevCov)
  Tracking_State_Update/3(trkID) -> Track_Association/3(trkID), TW_TrkID/1, Track_Update/3(pID)
  UD_ID/1 -> Tracking_State_Update/6(prevID)
  Tracking_State_Update/4(trkStatus) -> Track_Association/4(trkStatus), TW_TrkStatus/1, Track_Update/4(pStatus)
  UD_Status/1 -> Tracking_State_Update/7(prevStatus)
  Tracking_State_Update/5(nextID) -> TW_NextID/1, Track_Update/5(pNextID)
  UD_NextID/1 -> Tracking_State_Update/8(prevNextID)
  Tracking_State_Update/6(egoTransform) -> TW_EgoTransform/1, Track_Update/12(egoTransform)
  Tracking_State_Update/7(predDiag) -> TW_PredDiag/1
  Track_Association/1(trkAssign) -> TW_TrkAssign/1, Track_Update/9(trkAssign)
  Track_Association/2(numAssigned) -> TW_NumAssigned/1
  Track_Association/3(assocDiag) -> TW_AssocDiag/1
  UD_Hits/1 -> Track_Update/6(prevHits)
  UD_Tsu/1 -> Track_Update/7(prevTsu)
  UD_R1/1 -> Track_Update/8(prevR1)
  Track_Update/1(oState) -> TW_StatePost/1, Track_Lifecycle/1(iState)
  Track_Update/2(oCov) -> TW_CovPost/1, Track_Lifecycle/2(iCov)
  Track_Update/3(oID) -> TW_IDPost/1, Track_Lifecycle/3(iID)
  Track_Update/4(oStatus) -> TW_StatusPost/1, Track_Lifecycle/4(iStatus)
  Track_Update/5(oNextID) -> TW_NextIDPost/1, Track_Lifecycle/5(iNextID)
  Track_Update/6(oHits) -> TW_Hits/1, Track_Lifecycle/6(iHits)
  Track_Update/7(oTsu) -> TW_Tsu/1, Track_Lifecycle/7(iTsu)
  Track_Update/8(oR1) -> TW_R1/1, Track_Lifecycle/8(iR1)
  Track_Update/9(updDiag) -> TW_UpdDiag/1
  UD_Win/1 -> Track_Lifecycle/9(prevWin)
  UD_Age/1 -> Track_Lifecycle/10(prevAge)
  UD_Lost/1 -> Track_Lifecycle/11(prevLost)
  Track_Lifecycle/1(oState) -> UD_State/1, TW_StateLife/1, Track_History/1(trkState), Prediction_Horizons/1(trkState), TrackState/1
  Track_Lifecycle/2(oCov) -> UD_Cov/1, TW_CovLife/1, Prediction_Horizons/2(trkCov), TrackCov/1
  Track_Lifecycle/3(oID) -> UD_ID/1, TW_IDLife/1, Track_History/2(trkID), TrackID/1
  Track_Lifecycle/4(oStatus) -> UD_Status/1, TW_StatusLife/1, Track_History/3(trkStatus), Prediction_Horizons/3(trkStatus), TrackStatus/1
  Track_Lifecycle/5(oNextID) -> UD_NextID/1
  Track_Lifecycle/6(oHits) -> UD_Hits/1
  Track_Lifecycle/7(oTsu) -> UD_Tsu/1, Track_History/4(trkTsu)
  Track_Lifecycle/8(oR1) -> UD_R1/1
  Track_Lifecycle/9(oWin) -> UD_Win/1, TW_Win/1
  Track_Lifecycle/10(oAge) -> UD_Age/1, TW_Age/1
  Track_Lifecycle/11(oLost) -> UD_Lost/1, TW_Lost/1
  Track_Lifecycle/12(lifeDiag) -> TW_LifeDiag/1
  SimClock/1 -> Track_History/5(simTime)
  UD_Hist/1 -> Track_History/6(prevHist)
  UD_Ring/1 -> Track_History/7(prevRing)
  Track_History/1(hist) -> UD_Hist/1, TW_Hist/1
  Track_History/2(ringIdx) -> UD_Ring/1, TW_Ring/1
  Track_History/3(validCount) -> TW_VC/1
  Track_History/4(histSpan) -> TW_Span/1
  Prediction_Horizons/1(trkPred) -> TW_Pred/1
  Track_Update/10(oAttr) -> Track_Lifecycle/12(iAttr)
  Track_Lifecycle/13(oAttr) -> UD_Attr/1
  UD_Attr/1 -> Track_Update/13(prevAttr)
  Track_Lifecycle/14(oTrackAttributes) -> TW_TrackAttr/1, TrackAttributes/1

== system ADAS_Main/Vision_Perception ==
  Actors : Inport
  Vision Detection Generator : drivingscenarioandsensors/Vision Detection Generator  SensorIndex=1  DetectorOutput=Objects only  UpdateInterval=0.1  LaneUpdateInterval=0.1  SensorLocation=[ 1.9, 0 ]  Height=1.1  Yaw=0  Pitch=1  Roll=0  BusNameSource=Auto  BusName=BusObjectDetections  BusName2Source=Auto  BusName2=BusLaneDetections  MaxNumDetectionsSource=Property  MaxNumDetections=50  MaxNumLanesSource=Property  MaxNumLanes=30  DetectionCoordinates=Ego Cartesian  SimulateUsing=Interpreted execution  MaxRange=150  BoundingBoxAccuracy=5  ProcessNoiseIntensity=5  MaxSpeed=100  MaxAllowedOcclusion=0.5  MinObjectImageSize=[ 15, 15 ]  DetectionProbability=0.9  FalsePositivesPerImage=0.1  MinLaneImageSize=[ 20, 3 ]  LaneBoundaryAccuracy=3  HasNoise=on  InitialSeedSource=Repeatable  InitialSeed=0  UsedSeed=driving.internal.SimulinkUtilities.seedManager(gcb)  ActorProfilesSource=From Scenario Reader block  ActorProfilesParameters=driving.internal.ActorProfilesParameters  ActorProfilesExpression=struct( 'ClassID', 0, 'Length', 4.7, 'Width', 1.8, 'Height', 1.4, 'OriginOffset', [ -1.35, 0, 0 ] )  Intrinsics=driving.internal.cameraIntrinsics
  ObjectDetections : Outport
  wires:
  Actors/1 -> Vision Detection Generator/1
  Vision Detection Generator/1 -> ObjectDetections/1

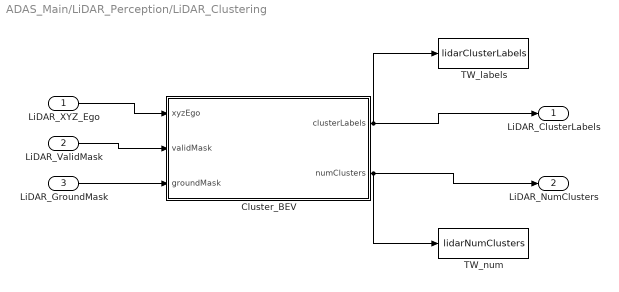
== system ADAS_Main/LiDAR_Perception/LiDAR_Clustering ==
  LiDAR_XYZ_Ego : Inport
  LiDAR_ValidMask : Inport  Port=2
  LiDAR_GroundMask : Inport  Port=3
  Cluster_BEV : MATLAB Function  TreatAsAtomicUnit=on
  TW_labels : ToWorkspace  VariableName=lidarClusterLabels  SaveFormat=Timeseries  SampleTime=-1
  TW_num : ToWorkspace  VariableName=lidarNumClusters  SaveFormat=Timeseries  SampleTime=-1
  LiDAR_ClusterLabels : Outport
  LiDAR_NumClusters : Outport  Port=2
  wires:
  LiDAR_XYZ_Ego/1 -> Cluster_BEV/1(xyzEgo)
  LiDAR_ValidMask/1 -> Cluster_BEV/2(validMask)
  LiDAR_GroundMask/1 -> Cluster_BEV/3(groundMask)
  Cluster_BEV/1(clusterLabels) -> LiDAR_ClusterLabels/1, TW_labels/1
  Cluster_BEV/2(numClusters) -> LiDAR_NumClusters/1, TW_num/1

== system ADAS_Main/LiDAR_Perception/LiDAR_Detection_Formatting ==
  LiDARFeatures : Inport
  LiDAR_NumClusters : Inport  Port=2
  Format_LiDAR_Detections : MATLAB Function  TreatAsAtomicUnit=on
  TW_det : ToWorkspace  VariableName=lidarDetections  SaveFormat=Timeseries  SampleTime=-1
  TW_num : ToWorkspace  VariableName=lidarNumDetections  SaveFormat=Timeseries  SampleTime=-1
  LiDARDetections : Outport
  NumLiDARDetections : Outport  Port=2
  wires:
  LiDARFeatures/1 -> Format_LiDAR_Detections/1(LiDARFeatures)
  LiDAR_NumClusters/1 -> Format_LiDAR_Detections/2(numClusters)
  Format_LiDAR_Detections/1(LiDARDetections) -> LiDARDetections/1, TW_det/1
  Format_LiDAR_Detections/2(NumLiDARDetections) -> NumLiDARDetections/1, TW_num/1

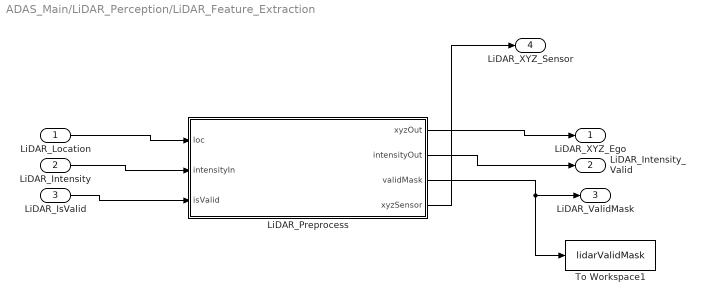
== system ADAS_Main/LiDAR_Perception/LiDAR_Feature_Extraction ==
  LiDAR_Location : Inport
  LiDAR_Intensity : Inport  Port=2
  LiDAR_IsValid : Inport  Port=3
  LiDAR_Preprocess : MATLAB Function  TreatAsAtomicUnit=on
  To Workspace1 : ToWorkspace  VariableName=lidarValidMask  SaveFormat=Timeseries  SampleTime=-1
  LiDAR_XYZ_Ego : Outport
  LiDAR_Intensity_Valid : Outport  Port=2
  LiDAR_ValidMask : Outport  Port=3
  LiDAR_XYZ_Sensor : Outport  Port=4
  wires:
  LiDAR_Location/1 -> LiDAR_Preprocess/1(loc)
  LiDAR_Intensity/1 -> LiDAR_Preprocess/2(intensityIn)
  LiDAR_IsValid/1 -> LiDAR_Preprocess/3(isValid)
  LiDAR_Preprocess/1(xyzOut) -> LiDAR_XYZ_Ego/1
  LiDAR_Preprocess/2(intensityOut) -> LiDAR_Intensity_Valid/1
  LiDAR_Preprocess/3(validMask) -> To Workspace1/1, LiDAR_ValidMask/1
  LiDAR_Preprocess/4(xyzSensor) -> LiDAR_XYZ_Sensor/1

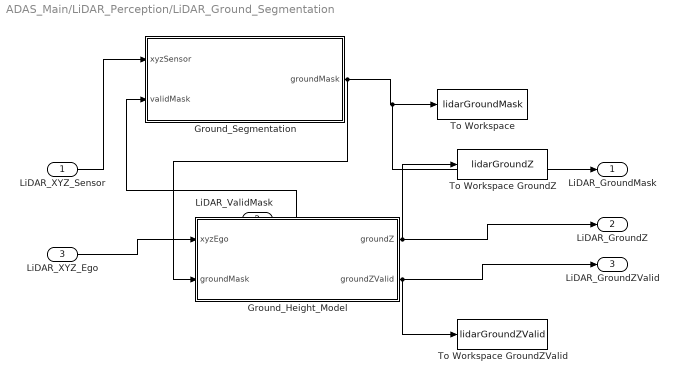
== system ADAS_Main/LiDAR_Perception/LiDAR_Ground_Segmentation ==
  LiDAR_XYZ_Sensor : Inport
  LiDAR_ValidMask : Inport  Port=2
  LiDAR_XYZ_Ego : Inport  Port=3
  Ground_Height_Model : MATLAB Function  TreatAsAtomicUnit=on
  Ground_Segmentation : MATLAB Function  TreatAsAtomicUnit=on
  To Workspace : ToWorkspace  VariableName=lidarGroundMask  SaveFormat=Timeseries  SampleTime=-1
  To Workspace GroundZ : ToWorkspace  VariableName=lidarGroundZ  SaveFormat=Timeseries  SampleTime=-1
  To Workspace GroundZValid : ToWorkspace  VariableName=lidarGroundZValid  SaveFormat=Timeseries  SampleTime=-1
  LiDAR_GroundMask : Outport
  LiDAR_GroundZ : Outport  Port=2
  LiDAR_GroundZValid : Outport  Port=3
  wires:
  LiDAR_XYZ_Sensor/1 -> Ground_Segmentation/1(xyzSensor)
  LiDAR_ValidMask/1 -> Ground_Segmentation/2(validMask)
  Ground_Segmentation/1(groundMask) -> LiDAR_GroundMask/1, To Workspace/1, Ground_Height_Model/2(groundMask)
  LiDAR_XYZ_Ego/1 -> Ground_Height_Model/1(xyzEgo)
  Ground_Height_Model/1(groundZ) -> LiDAR_GroundZ/1, To Workspace GroundZ/1
  Ground_Height_Model/2(groundZValid) -> LiDAR_GroundZValid/1, To Workspace GroundZValid/1

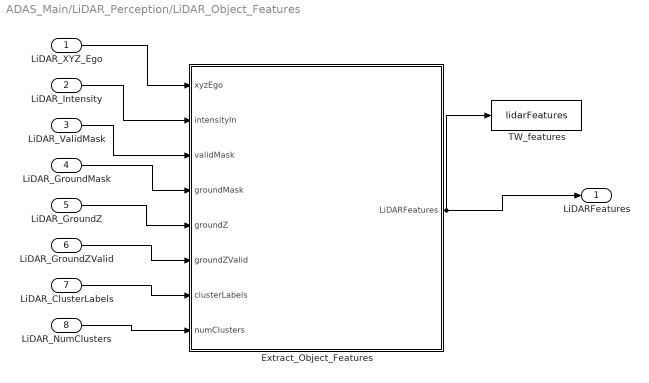
== system ADAS_Main/LiDAR_Perception/LiDAR_Object_Features ==
  LiDAR_XYZ_Ego : Inport
  LiDAR_Intensity : Inport  Port=2
  LiDAR_ValidMask : Inport  Port=3
  LiDAR_GroundMask : Inport  Port=4
  LiDAR_GroundZ : Inport  Port=5
  LiDAR_GroundZValid : Inport  Port=6
  LiDAR_ClusterLabels : Inport  Port=7
  LiDAR_NumClusters : Inport  Port=8
  Extract_Object_Features : MATLAB Function  TreatAsAtomicUnit=on
  TW_features : ToWorkspace  VariableName=lidarFeatures  SaveFormat=Timeseries  SampleTime=-1
  LiDARFeatures : Outport
  wires:
  LiDAR_XYZ_Ego/1 -> Extract_Object_Features/1(xyzEgo)
  LiDAR_Intensity/1 -> Extract_Object_Features/2(intensityIn)
  LiDAR_ValidMask/1 -> Extract_Object_Features/3(validMask)
  LiDAR_GroundMask/1 -> Extract_Object_Features/4(groundMask)
  LiDAR_GroundZ/1 -> Extract_Object_Features/5(groundZ)
  LiDAR_GroundZValid/1 -> Extract_Object_Features/6(groundZValid)
  LiDAR_ClusterLabels/1 -> Extract_Object_Features/7(clusterLabels)
  LiDAR_NumClusters/1 -> Extract_Object_Features/8(numClusters)
  Extract_Object_Features/1(LiDARFeatures) -> LiDARFeatures/1, TW_features/1

== system ADAS_Main/Radar_Perception/Radar_Feature_Extraction ==
  RawRadarDetections : Inport
  Extract_Radar_Features : MATLAB Function  TreatAsAtomicUnit=on
  EnhancedRadar : Outport
  RadarFeatures : Outport  Port=2
  wires:
  RawRadarDetections/1 -> Extract_Radar_Features/1(u), EnhancedRadar/1
  Extract_Radar_Features/1(RadarFeatures) -> RadarFeatures/1
